simulink model "HIRES_sim"  (Simulink 7.4)
settings: Solver=ode15s  StartTime=0.0  StopTime=321.81220  RelTol=1e-3
settings Model: Creator=David  LastModifiedBy=David
settings SolverCC: SolverResetMethod=Robust
settings DebuggingCC: StrictBusMsg=ErrorLevel1

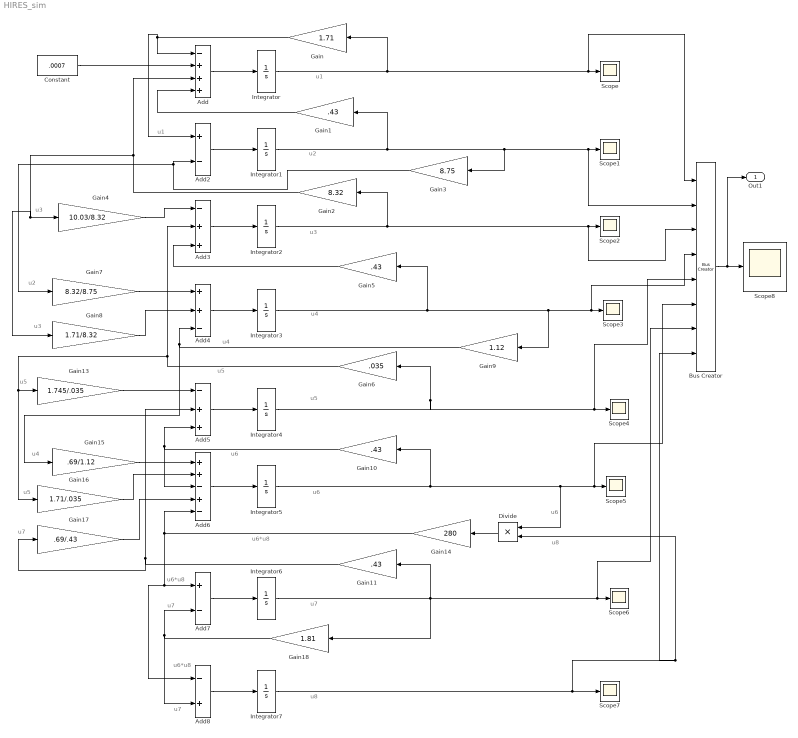
== system HIRES_sim ==
  note: u1
  note: u2
  note: u3
  note: u4
  note: u1
  note: u5
  note: u2
  note: u3
  note: u3
  note: u7
  note: u8
  note: u6
  note: u8
  note: u6
  note: u5
  note: u5
  note: u4
  note: u4
  note: u5
  note: u6
  note: u7
  note: u6*u8
  note: u6*u8
  note: u7
  note: u7
  note: u6*u8
  Add : Sum  Inputs=-+++  OutDataType=fixdt(1, 16)  OutScaling=2^-10
  Add2 : Sum  Inputs=+-  OutDataType=fixdt(1, 16)  OutScaling=2^-10
  Add3 : Sum  Inputs=-++  OutDataType=fixdt(1, 16)  OutScaling=2^-10
  Add4 : Sum  Inputs=++-  OutDataType=fixdt(1, 16)  OutScaling=2^-10
  Add5 : Sum  Inputs=-++  OutDataType=fixdt(1, 16)  OutScaling=2^-10
  Add6 : Sum  Inputs=++-+-  OutDataType=fixdt(1, 16)  OutScaling=2^-10
  Add7 : Sum  Inputs=+-  OutDataType=fixdt(1, 16)  OutScaling=2^-10
  Add8 : Sum  Inputs=-+  OutDataType=fixdt(1, 16)  OutScaling=2^-10
  Bus Creator : BusCreator  Inputs=8
  Constant : Constant  Value=.0007  OutDataType=fixdt(1, 16)  OutScaling=2^0
  Divide : Product  Inputs=**  OutDataType=fixdt(1, 16)  OutScaling=2^-10
  Gain : Gain  Gain=1.71  ParameterDataType=fixdt(1, 16)  ParameterScaling=2^0  OutDataType=fixdt(1, 16)  OutScaling=2^0
  Gain{1,5,10..11} (4 alike) : Gain  Gain=.43  ParameterDataType=fixdt(1, 16)  ParameterScaling=2^0  OutDataType=fixdt(1, 16)  OutScaling=2^0
  Gain13 : Gain  Gain=1.745/.035  ParameterDataType=fixdt(1, 16)  ParameterScaling=2^0  OutDataType=fixdt(1, 16)  OutScaling=2^0
  Gain14 : Gain  Gain=280  ParameterDataType=fixdt(1, 16)  ParameterScaling=2^0  OutDataType=fixdt(1, 16)  OutScaling=2^0
  Gain15 : Gain  Gain=.69/1.12  ParameterDataType=fixdt(1, 16)  ParameterScaling=2^0  OutDataType=fixdt(1, 16)  OutScaling=2^0
  Gain16 : Gain  Gain=1.71/.035  ParameterDataType=fixdt(1, 16)  ParameterScaling=2^0  OutDataType=fixdt(1, 16)  OutScaling=2^0
  Gain17 : Gain  Gain=.69/.43  ParameterDataType=fixdt(1, 16)  ParameterScaling=2^0  OutDataType=fixdt(1, 16)  OutScaling=2^0
  Gain18 : Gain  Gain=1.81  ParameterDataType=fixdt(1, 16)  ParameterScaling=2^0  OutDataType=fixdt(1, 16)  OutScaling=2^0
  Gain2 : Gain  Gain=8.32  ParameterDataType=fixdt(1, 16)  ParameterScaling=2^0  OutDataType=fixdt(1, 16)  OutScaling=2^0
  Gain3 : Gain  Gain=8.75  ParameterDataType=fixdt(1, 16)  ParameterScaling=2^0  OutDataType=fixdt(1, 16)  OutScaling=2^0
  Gain4 : Gain  Gain=10.03/8.32  ParameterDataType=fixdt(1, 16)  ParameterScaling=2^0  OutDataType=fixdt(1, 16)  OutScaling=2^0
  Gain6 : Gain  Gain=.035  ParameterDataType=fixdt(1, 16)  ParameterScaling=2^0  OutDataType=fixdt(1, 16)  OutScaling=2^0
  Gain7 : Gain  Gain=8.32/8.75  ParameterDataType=fixdt(1, 16)  ParameterScaling=2^0  OutDataType=fixdt(1, 16)  OutScaling=2^0
  Gain8 : Gain  Gain=1.71/8.32  ParameterDataType=fixdt(1, 16)  ParameterScaling=2^0  OutDataType=fixdt(1, 16)  OutScaling=2^0
  Gain9 : Gain  Gain=1.12  ParameterDataType=fixdt(1, 16)  ParameterScaling=2^0  OutDataType=fixdt(1, 16)  OutScaling=2^0
  Integrator : Integrator  InitialCondition=1
  Integrator{1..6} (6 alike) : Integrator
  Integrator7 : Integrator  InitialCondition=.0057
  Scope{,1..8} (9 alike) : Scope
      Scope2 settings: SaveName=ScopeData2
      Scope3 settings: SaveName=ScopeData3
      Scope4 settings: SaveName=ScopeData4
      Scope5 settings: SaveName=ScopeData5
      Scope6 settings: SaveName=ScopeData6
      Scope7 settings: SaveName=ScopeData7
      Scope8 settings: SaveName=ScopeData8
  Out1 : Outport  OutDataType=fixdt(1, 16)  OutScaling=2^0
  wires:
  Integrator/1 -> Gain/1, Scope/1, Bus Creator/1
  Constant/1 -> Add/2
  Gain/1 -> Add/1, Add2/1
  Add/1 -> Integrator/1
  Add2/1 -> Integrator1/1
  Integrator1/1 -> Gain1/1, Gain3/1, Scope1/1, Bus Creator/2
  Gain1/1 -> Add/4
  Add3/1 -> Integrator2/1
  Integrator2/1 -> Gain2/1, Scope2/1, Bus Creator/3
  Gain2/1 -> Add/3, Gain4/1, Gain8/1
  Add4/1 -> Integrator3/1
  Integrator3/1 -> Gain5/1, Gain9/1, Scope3/1, Bus Creator/4
  Gain3/1 -> Add2/2, Gain7/1
  Gain4/1 -> Add3/1
  Gain5/1 -> Add3/3
  Add5/1 -> Integrator4/1
  Integrator4/1 -> Gain6/1, Scope4/1, Bus Creator/5
  Gain6/1 -> Add3/2, Gain13/1, Gain16/1
  Gain7/1 -> Add4/1
  Gain8/1 -> Add4/2
  Gain9/1 -> Add4/3, Gain15/1
  Add6/1 -> Integrator5/1
  Integrator5/1 -> Gain10/1, Divide/1, Scope5/1, Bus Creator/6
  Add7/1 -> Integrator6/1
  Integrator6/1 -> Gain11/1, Gain18/1, Scope6/1, Bus Creator/7
  Add8/1 -> Integrator7/1
  Integrator7/1 -> Scope7/1, Divide/2, Bus Creator/8
  Gain13/1 -> Add5/1
  Gain10/1 -> Add5/3, Add6/3
  Gain11/1 -> Add5/2, Gain17/1
  Divide/1 -> Gain14/1
  Gain14/1 -> Add6/5, Add7/1, Add8/1
  Gain15/1 -> Add6/1
  Gain16/1 -> Add6/2
  Gain17/1 -> Add6/4
  Gain18/1 -> Add7/2, Add8/2
  Bus Creator/1 -> Scope8/1, Out1/1
